simulink model "fusionS_22a1"  (R2022a)
settings: Solver=VariableStepAuto  StartTime=0.0  StopTime=10.0  RelTol=1e-3
values from neighbouring files (symbols this model uses):
  covA = 800    [fusion_parameters.m]
  covG = 0.0001    [fusion_parameters.m]
  covM = 80    [fusion_parameters.m]
  covP = 34    [fusion_parameters.m]
  covV = 0.0464    [fusion_parameters.m]
  initstate = zeros(28,1)    [fusion_parameters.m]
undefined symbols (not defined in the file or in its folder): acceleration, angularVelocity, MagneticField, position, rateImu, ratioGps, ratioMag, velocity
settings Model: Creator=fullb  LastModifiedBy=Inver
settings ModelReferenceCC: EnableRefExpFcnMdlSchedulingChecks=off
settings RTWCC: Description=Generic Real-Time Target

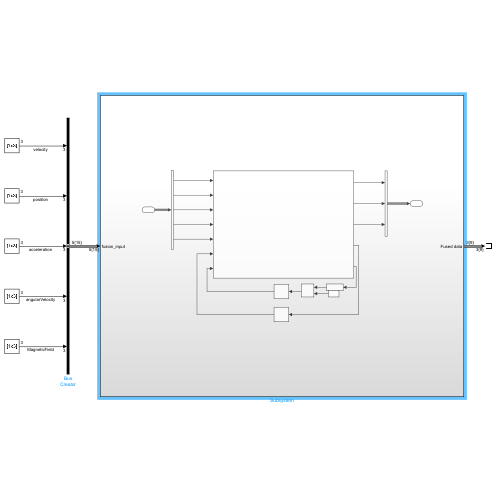
[thumbnail: Simulink's stored preview of the top-level diagram]
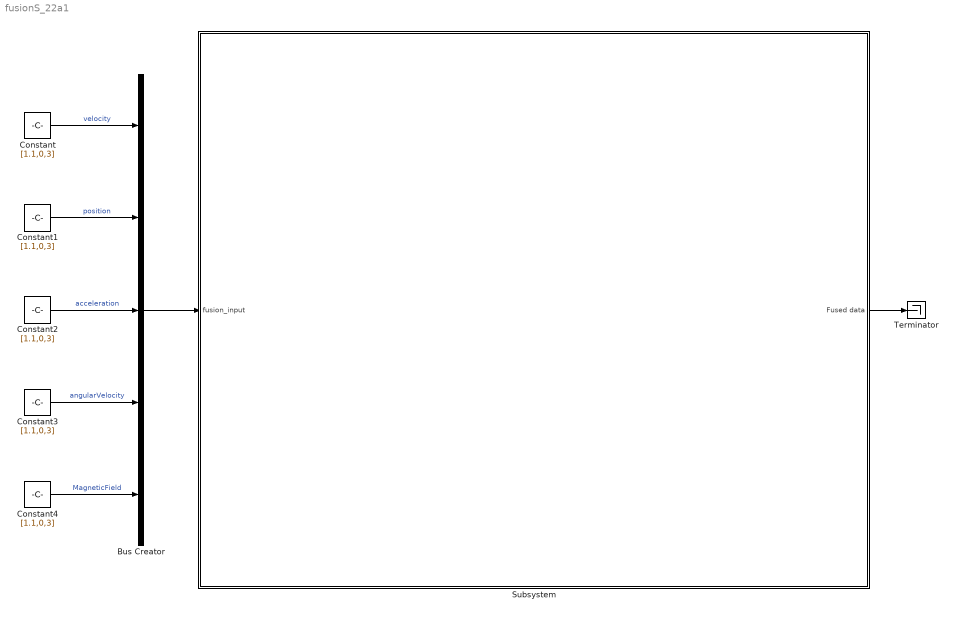
== system fusionS_22a1 ==
  Bus Creator : BusCreator  Inputs=velocity,position,acceleration,angularVelocity,MagneticField
  Constant{,1..4} (5 alike) : Constant  Value=[1.1,0,3]
  Subsystem : Subsystem
  Terminator : Terminator
  wires:
  Bus Creator/1 -> Subsystem/1(fusion_input)
  Subsystem/1(Fused data) -> Terminator/1
  Constant/1 -> Bus Creator/1  "velocity"
  Constant1/1 -> Bus Creator/2  "position"
  Constant2/1 -> Bus Creator/3  "acceleration"
  Constant3/1 -> Bus Creator/4  "angularVelocity"
  Constant4/1 -> Bus Creator/5  "MagneticField"

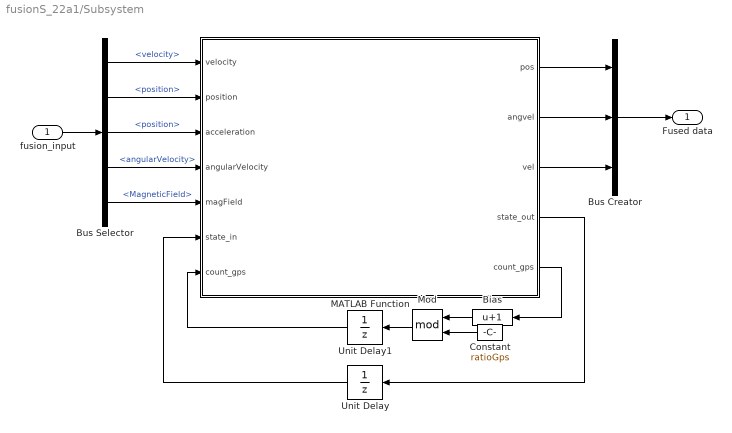
== system fusionS_22a1/Subsystem ==
  fusion_input : Inport
  Bias : Bias  Bias=1  SaturateOnIntegerOverflow=off
  Bus Creator : BusCreator  Inputs=3
  Bus Selector : BusSelector  OutputSignals=velocity,position,position,angularVelocity,MagneticField
  Constant : Constant  Value=ratioGps
  MATLAB Function : MATLAB Function  TreatAsAtomicUnit=on
  Mod : Math  Operator=mod
  Unit Delay : UnitDelay  InitialCondition=initstate  SampleTime=t  HasFrameUpgradeWarning=on
  Unit Delay1 : UnitDelay  SampleTime=t  HasFrameUpgradeWarning=on
  Fused data : Outport
  wires:
  Bus Selector/1 -> MATLAB Function/1(velocity)  "<velocity>"
  Bus Selector/4 -> MATLAB Function/4(angularVelocity)  "<angularVelocity>"
  Unit Delay/1 -> MATLAB Function/6(state_in)
  MATLAB Function/5(count_gps) -> Bias/1
  Unit Delay1/1 -> MATLAB Function/7("count_gps ")
  MATLAB Function/4(state_out) -> Unit Delay/1
  Bus Selector/2 -> MATLAB Function/2(position)  "<position>"
  Bus Selector/3 -> MATLAB Function/3(acceleration)  "<position>"
  fusion_input/1 -> Bus Selector/1
  Bus Selector/5 -> MATLAB Function/5(magField)  "<MagneticField>"
  MATLAB Function/1(pos) -> Bus Creator/1
  MATLAB Function/2(angvel) -> Bus Creator/2
  MATLAB Function/3(vel) -> Bus Creator/3
  Bus Creator/1 -> Fused data/1
  Mod/1 -> Unit Delay1/1
  Bias/1 -> Mod/1
  Constant/1 -> Mod/2

== matlab function fusionS_22a1/Subsystem/MATLAB Function ==
  data: pos output; angvel output size=[1,3]; velocity input size=[1,3]; vel output size=[1,3]; state_out output; position input size=[1,3]; acceleration input size=[1,3]; angularVelocity input size=[1,3]; magField input size=[1,3]; state_in input; count_gps input; count_gps output; covG parameter; covA parameter; covM parameter; covP parameter; covV parameter; ratioGps parameter; ratioMag parameter; rateImu parameter
function [pos,angvel,vel, state_out, count_gps] = fusion(velocity, position ,acceleration,angularVelocity, magField,state_in,count_gps, covG, covA, covM, covP, covV, ratioGps, ratioMag, rateImu) 

%creating the filter and loading previous state 
filter = insfilterAsync();
filter.State= state_in;
filter.predict((1/rateImu));

%the actual fusion
fuseaccel(filter,acceleration,covA);
fusegyro(filter,angularVelocity,covG);

%check for frequency of magnetometer if not do the same as for the gps using ratioMag 
fusemag(filter, magField,covM);

%if ~mod(count,ratioGps)
if ~count_gps
    fusegps(filter,position,covP,velocity,covV);
end
[pos,angvel1,vel] = pose(filter);

angvel = euler(angvel1,"ZYX","Frame");

% update filter state
state_out = filter.State;

end
